simulink model "ff22_f22"  (R2015b)
settings: Solver=VariableStepAuto  StartTime=0.0  StopTime=10.0  RelTol=1e-3
undefined symbols (not defined in the file): a, b, c, Csfl, Csfr, Csrl, Csrr, d, Ixx, Ksfl, Ksfr, Ksrl, Ksrr, S
settings Model: Creator=Guest  LastModifiedBy=Guest

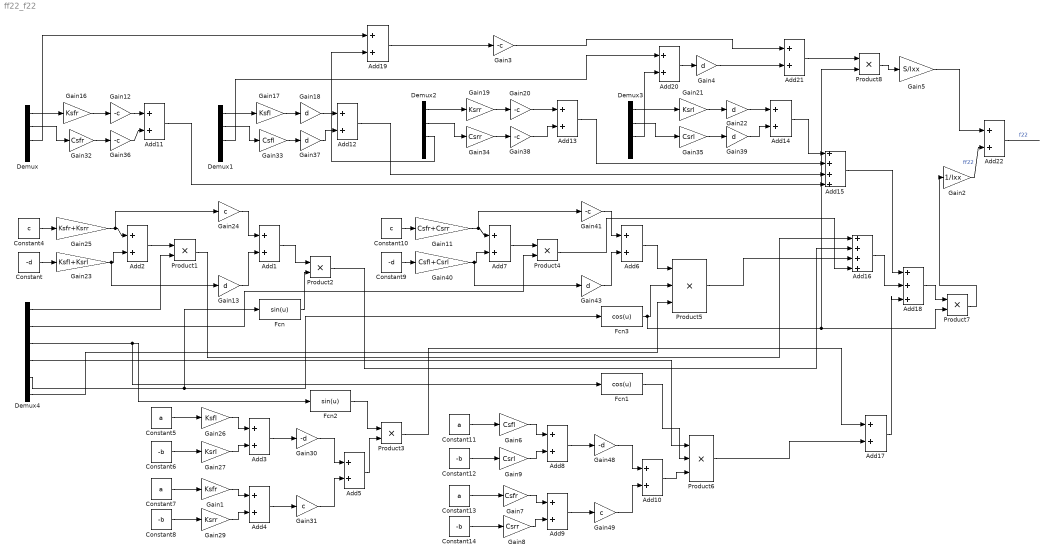
== system ff22_f22 ==
  Add{1..14,17,19..22} (19 alike) : Sum
  Add15 : Sum  Inputs=++++
  Add16 : Sum  Inputs=++++
  Add18 : Sum  Inputs=+++
  Constant : Constant  Value=-d
  Constant10 : Constant  Value=c
  Constant{5,7,11,13} (4 alike) : Constant  Value=a
  Constant{6,8,12,14} (4 alike) : Constant  Value=-b
  Constant4 : Constant  Value=c
  Constant9 : Constant  Value=-d
  Demux{,1..3} (4 alike) : Demux
  Demux4 : Demux  Outputs=6
  Fcn : Fcn  Expr=sin(u)
  Fcn1 : Fcn  Expr=cos(u)
  Fcn2 : Fcn  Expr=sin(u)
  Fcn3 : Fcn  Expr=cos(u)
  Gain1 : Gain  Gain=Ksfr
  Gain11 : Gain  Gain=Csfr+Csrr
  Gain{3,12,20,36,38,41} (6 alike) : Gain  Gain=-c
  Gain{4,13,18,22,37,39,43} (7 alike) : Gain  Gain=d
  Gain16 : Gain  Gain=Ksfr
  Gain17 : Gain  Gain=Ksfl
  Gain19 : Gain  Gain=Ksrr
  Gain2 : Gain  Gain=1/Ixx
  Gain21 : Gain  Gain=Ksrl
  Gain23 : Gain  Gain=Ksfl+Ksrl
  Gain24 : Gain  Gain=c
  Gain25 : Gain  Gain=Ksfr+Ksrr
  Gain26 : Gain  Gain=Ksfl
  Gain27 : Gain  Gain=Ksrl
  Gain29 : Gain  Gain=Ksrr
  Gain30 : Gain  Gain=-d
  Gain31 : Gain  Gain=c
  Gain32 : Gain  Gain=Csfr
  Gain33 : Gain  Gain=Csfl
  Gain34 : Gain  Gain=Csrr
  Gain35 : Gain  Gain=Csrl
  Gain40 : Gain  Gain=Csfl+Csrl
  Gain48 : Gain  Gain=-d
  Gain49 : Gain  Gain=c
  Gain5 : Gain  Gain=S/Ixx
  Gain6 : Gain  Gain=Csfl
  Gain7 : Gain  Gain=Csfr
  Gain8 : Gain  Gain=Csrr
  Gain9 : Gain  Gain=Csrl
  Product{1..4,7..8} (6 alike) : Product
  Product5 : Product  Inputs=3
  Product6 : Product  Inputs=3
  wires:
  Demux/1 -> Gain16/1
  Gain16/1 -> Gain12/1
  Demux1/1 -> Gain17/1
  Gain17/1 -> Gain18/1
  Demux2/1 -> Gain19/1
  Gain19/1 -> Gain20/1
  Demux3/1 -> Gain21/1
  Gain21/1 -> Gain22/1
  Constant/1 -> Gain23/1
  Constant4/1 -> Gain25/1
  Gain23/1 -> Gain13/1, Add2/2
  Gain25/1 -> Gain24/1, Add2/1
  Add2/1 -> Product1/1
  Demux4/1 -> Product1/2
  Gain24/1 -> Add1/1
  Gain13/1 -> Add1/2
  Constant5/1 -> Gain26/1
  Constant6/1 -> Gain27/1
  Gain26/1 -> Add3/1
  Gain27/1 -> Add3/2
  Constant8/1 -> Gain29/1
  Constant7/1 -> Gain1/1
  Gain1/1 -> Add4/1
  Gain29/1 -> Add4/2
  Add3/1 -> Gain30/1
  Add4/1 -> Gain31/1
  Demux4/3 -> Fcn1/1, Fcn2/1
  Add1/1 -> Product2/1
  Fcn/1 -> Product2/2
  Demux4/5 -> Fcn/1, Fcn3/1
  Gain30/1 -> Add5/1
  Gain31/1 -> Add5/2
  Add5/1 -> Product3/2
  Fcn2/1 -> Product3/1
  Demux/2 -> Gain32/1
  Demux1/2 -> Gain33/1
  Demux2/2 -> Gain34/1
  Demux3/2 -> Gain35/1
  Gain32/1 -> Gain36/1
  Gain33/1 -> Gain37/1
  Gain34/1 -> Gain38/1
  Gain35/1 -> Gain39/1
  Constant10/1 -> Gain11/1
  Gain40/1 -> Gain43/1, Add7/2
  Gain11/1 -> Add7/1, Gain41/1
  Add7/1 -> Product4/1
  Demux4/2 -> Product4/2
  Gain41/1 -> Add6/1
  Gain43/1 -> Add6/2
  Add6/1 -> Product5/1
  Constant9/1 -> Gain40/1
  Fcn3/1 -> Product8/2, Product7/2, Product5/2
  Constant11/1 -> Gain6/1
  Constant12/1 -> Gain9/1
  Gain6/1 -> Add8/1
  Gain9/1 -> Add8/2
  Constant14/1 -> Gain8/1
  Constant13/1 -> Gain7/1
  Gain7/1 -> Add9/1
  Add8/1 -> Gain48/1
  Add9/1 -> Gain49/1
  Gain48/1 -> Add10/1
  Gain49/1 -> Add10/2
  Add10/1 -> Product6/3
  Fcn1/1 -> Product6/2
  Gain8/1 -> Add9/2
  Demux4/6 -> Product5/3
  Gain12/1 -> Add11/1
  Gain36/1 -> Add11/2
  Gain18/1 -> Add12/1
  Gain37/1 -> Add12/2
  Gain20/1 -> Add13/1
  Gain38/1 -> Add13/2
  Gain22/1 -> Add14/1
  Gain39/1 -> Add14/2
  Add14/1 -> Add15/1
  Add13/1 -> Add15/2
  Add12/1 -> Add15/3
  Add11/1 -> Add15/4
  Product1/1 -> Add16/1
  Product2/1 -> Add16/2
  Product5/1 -> Add16/3
  Product4/1 -> Add16/4
  Product3/1 -> Add17/1
  Product6/1 -> Add17/2
  Add15/1 -> Add18/1
  Add17/1 -> Add18/3
  Add16/1 -> Add18/2
  Add18/1 -> Product7/1
  Product7/1 -> Gain2/1
  Demux/3 -> Add19/1
  Add19/1 -> Gain3/1
  Add20/1 -> Gain4/1
  Gain4/1 -> Add21/2
  Gain3/1 -> Add21/1
  Add21/1 -> Product8/1
  Product8/1 -> Gain5/1
  Gain5/1 -> Add22/1
  Gain2/1 -> Add22/2  "ff22"
  Add22/1 -> ?  "f22"
  Demux4/4 -> Product6/1
  Demux2/3 -> Add19/2
  Demux1/3 -> Add20/1
  Demux3/3 -> Add20/2
